simulink model "SLIPquadtrot"  (R2016a)
settings: Solver=ode45  StartTime=0.0  StopTime=10  MaxStep=1e-3  RelTol=1e-4  AbsTol=1e-6
values from neighbouring files (symbols this model uses):
  g = 9.81    [SLIPquad_params - Copy.m]    (also in SLIPquad_params.m; SLIPquad_paramswalk.m; purecmaes.m; purecmaeswalk.m)
  J = 4.58    [SLIPquad_params - Copy.m]    (also in SLIPquad_params.m; SLIPquad_paramswalk.m; purecmaes.m; purecmaeswalk.m)
  L = 0.5    [SLIPquad_params - Copy.m]    (also in SLIPquad_params.m; SLIPquad_paramswalk.m; purecmaes.m; purecmaeswalk.m)
  l0 = 1    [SLIPquad_params - Copy.m]    (also in SLIPquad_params.m; SLIPquad_paramswalk.m; purecmaes.m; purecmaeswalk.m)
  m = 80    [SLIPquad_params - Copy.m]    (also in SLIPquad_params.m; SLIPquad_paramswalk.m; purecmaes.m; purecmaeswalk.m)
  x0 = 0    [SLIPquad_params - Copy.m]    (also in SLIPquad_params.m; SLIPquad_paramswalk.m; purecmaes.m; purecmaeswalk.m)
  xrb0 = -l0*cos(a0br) + L*cos(t0)    [SLIPquad_params - Copy.m]    (also in SLIPquad_params.m)
  xrf0 = -l0*cos(a0fr) - L*cos(t0)    [SLIPquad_params - Copy.m]    (also in SLIPquad_params.m)
  y0 = 0.9730    (= 0.973)    [SLIPquad_params - Copy.m]    (also in SLIPquad_params.m = 0.9571; SLIPquad_paramswalk.m = x(6); purecmaes.m = 1; purecmaeswalk.m = x(6))
  yrb0 = l0*sin(a0br) + L*sin(t0)    [SLIPquad_params - Copy.m]    (also in SLIPquad_params.m)
  yrf0 = l0*sin(a0fr) - L*sin(t0)    [SLIPquad_params - Copy.m]    (also in SLIPquad_params.m)
libraries: simulink_extras x4, dspswit3 x1
settings Model: Creator=hgeyer  LastModifiedBy=Joe
settings DataIOCC: SaveFormat=Array  SignalLoggingSaveFormat=ModelDataLogs
settings OptimizationCC: ExpressionDepthLimit=2147483647
settings DebuggingCC: UnderspecifiedInitializationDetection=Classic  MergeDetectMultiDrivingBlocksExec=none  SolverPrmCheckMsg=warning  FcnCallInpInsideContextMsg=EnableAllAsWarning  AllowSymbolicDim=off  StateNameClashWarn=warning
settings HardwareCC: ProdBitPerPointer=32  ProdLargestAtomicFloat=None  ProdIntDivRoundTo=Undefined  ProdEndianess=Unspecified  ProdWordSize=32  ProdHWDeviceType=32-bit Generic
settings ModelReferenceCC: PropagateSignalLabelsOutOfModel=off
settings ConfigComp: CovModelRefEnable=Off

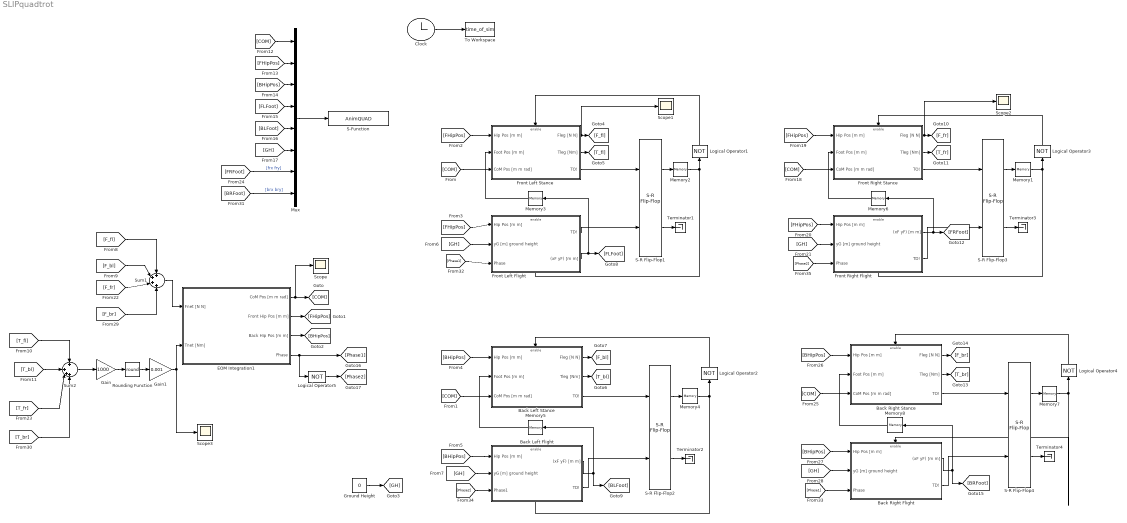
== system SLIPquadtrot ==
  Back Left Flight : Subsystem
  Back Left Stance : Subsystem
  Back Right Flight : Subsystem
  Back Right Stance : Subsystem
  Clock : Clock
      settings: Decimation=100
  EOM Integration1 : Subsystem
  Front Left Flight : Subsystem
  Front Left Stance : Subsystem
  Front Right Flight : Subsystem
  Front Right Stance : Subsystem
  Gain : Gain  Gain=1000
  Gain1 : Gain  Gain=0.001
  Ground Height : Constant  Value=0
  Logical Operator{1..5} (5 alike) : Logic  Operator=NOT  AllPortsSameDT=off  OutDataTypeStr=boolean
  Memory{1..2,4,7} (4 alike) : Memory  X0=1
  Memory3 : Memory  X0=[(x0 - xrf0) (y0 - yrf0) ]
  Memory5 : Memory  X0=[(x0 - xrb0) (y0 - yrb0)]
  Memory6 : Memory  X0=[(x0 - xrf0) (y0 - yrf0) ]
  Memory8 : Memory  X0=[(x0 - xrb0) (y0 - yrb0)]
  Mux : Mux  Inputs=8
  Rounding Function : Rounding  Operator=round
  S-Function : S-Function  FunctionName=AnimQUAD  Parameters=0.005  SFunctionDeploymentMode=off  EnableBusSupport=off
  S-R Flip-Flop{1..4} (4 alike) : simulink_extras/Flip Flops/S-R Flip-Flop  initial_condition=1
  Scope{,1..3} (4 alike) : Scope
  Sum1 : Sum  Inputs=++++
  Sum2 : Sum  Inputs=+|+++
  Terminator{1..4} (4 alike) : Terminator
  To Workspace : ToWorkspace  VariableName=time_of_sim  SampleTime=-1
      settings: MaxDataPoints=1
  wires:
  Front Left Stance/3(TO!) -> S-R Flip-Flop1/1
  S-R Flip-Flop1/1 -> Memory2/1
  Front Left Flight/1(TD!) -> S-R Flip-Flop1/2
  Memory2/1 -> Front Left Flight/Enable, Logical Operator1/1
  Logical Operator1/1 -> Front Left Stance/Enable
  S-R Flip-Flop1/2 -> Terminator1/1
  Front Left Flight/2((xF yF) [m m]) -> [FLFoot], Memory3/1
  Memory3/1 -> Front Left Stance/2(Foot Pos [m m])
  Back Left Stance/3(TO!) -> S-R Flip-Flop2/1
  S-R Flip-Flop2/1 -> Memory4/1
  Back Left Flight/2(TD!) -> S-R Flip-Flop2/2
  Memory4/1 -> Back Left Flight/Enable, Logical Operator2/1
  Logical Operator2/1 -> Back Left Stance/Enable
  S-R Flip-Flop2/2 -> Terminator2/1
  [GH] -> Back Left Flight/2(yG [m] ground height)
  Back Left Flight/1((xF yF) [m m]) -> [BLFoot], Memory5/1
  Memory5/1 -> Back Left Stance/2(Foot Pos [m m])
  Ground Height/1 -> [GH]
  [GH] -> Front Left Flight/2(yG [m] ground height)
  Front Left Stance/1(Fleg [N N]) -> Scope1/1, [F_fl]
  Front Left Stance/2(Tleg [Nm]) -> [T_fl]
  Back Left Stance/1(Fleg [N N]) -> [F_bl]
  Back Left Stance/2(Tleg [Nm]) -> [T_bl]
  [F_fl] -> Sum1/1
  [F_bl] -> Sum1/2
  [T_fl] -> Sum2/1
  [T_bl] -> Sum2/2
  Sum1/1 -> EOM Integration1/1(Fnet [N N])
  EOM Integration1/1(CoM Pos [m m rad]) -> Scope/1, [COM]
  EOM Integration1/2(Front Hip Pos [m m]) -> [FHipPos]
  EOM Integration1/3(Back Hip Pos [m m]) -> [BHipPos]
  [FHipPos] -> Front Left Stance/1(Hip Pos [m m])
  [FHipPos] -> Front Left Flight/1(Hip Pos [m m])
  [BHipPos] -> Back Left Stance/1(Hip Pos [m m])
  [BHipPos] -> Back Left Flight/1(Hip Pos [m m])
  [COM] -> Front Left Stance/3(CoM Pos [m m rad])
  [COM] -> Back Left Stance/3(CoM Pos [m m rad])
  Sum2/1 -> Gain/1
  Gain1/1 -> Scope3/1, EOM Integration1/2(Tnet [Nm])
  Gain/1 -> Rounding Function/1
  Rounding Function/1 -> Gain1/1
  Mux/1 -> S-Function/1
  [COM] -> Mux/1
  [FHipPos] -> Mux/2
  [BHipPos] -> Mux/3
  [FLFoot] -> Mux/4
  [BLFoot] -> Mux/5
  [GH] -> Mux/6
  [FRFoot] -> Mux/7  "[frx fry]"
  [BRFoot] -> Mux/8  "[brx bry]"
  Front Right Stance/3(TO!) -> S-R Flip-Flop3/1
  S-R Flip-Flop3/1 -> Memory1/1
  Front Right Flight/2(TD!) -> S-R Flip-Flop3/2
  Memory1/1 -> Front Right Flight/Enable, Logical Operator3/1
  Logical Operator3/1 -> Front Right Stance/Enable
  S-R Flip-Flop3/2 -> Terminator3/1
  Front Right Flight/1((xF yF) [m m]) -> Memory6/1, [FRFoot]
  Memory6/1 -> Front Right Stance/2(Foot Pos [m m])
  [GH] -> Front Right Flight/2(yG [m] ground height)
  Front Right Stance/1(Fleg [N N]) -> Scope2/1, [F_fr]
  Front Right Stance/2(Tleg [Nm]) -> [T_fr]
  [FHipPos] -> Front Right Stance/1(Hip Pos [m m])
  [FHipPos] -> Front Right Flight/1(Hip Pos [m m])
  [COM] -> Front Right Stance/3(CoM Pos [m m rad])
  [F_fr] -> Sum1/3
  [T_fr] -> Sum2/3
  Back Right Stance/3(TO!) -> S-R Flip-Flop4/1
  S-R Flip-Flop4/1 -> Memory7/1
  Back Right Flight/2(TD!) -> S-R Flip-Flop4/2
  Memory7/1 -> Back Right Flight/Enable, Logical Operator4/1
  Logical Operator4/1 -> Back Right Stance/Enable
  S-R Flip-Flop4/2 -> Terminator4/1
  [GH] -> Back Right Flight/2(yG [m] ground height)
  Back Right Flight/1((xF yF) [m m]) -> [BRFoot], Memory8/1
  Memory8/1 -> Back Right Stance/2(Foot Pos [m m])
  Back Right Stance/1(Fleg [N N]) -> [F_br]
  Back Right Stance/2(Tleg [Nm]) -> [T_br]
  [BHipPos] -> Back Right Stance/1(Hip Pos [m m])
  [BHipPos] -> Back Right Flight/1(Hip Pos [m m])
  [COM] -> Back Right Stance/3(CoM Pos [m m rad])
  [F_br] -> Sum1/4
  [T_br] -> Sum2/4
  Clock/1 -> To Workspace/1
  EOM Integration1/4(Phase) -> Logical Operator5/1, [Phase1]
  Logical Operator5/1 -> [Phase2]
  [Phase1] -> Front Left Flight/3(Phase)
  [Phase1] -> Back Right Flight/3(Phase)
  [Phase2] -> Back Left Flight/3(Phase1)
  [Phase2] -> Front Right Flight/3(Phase)

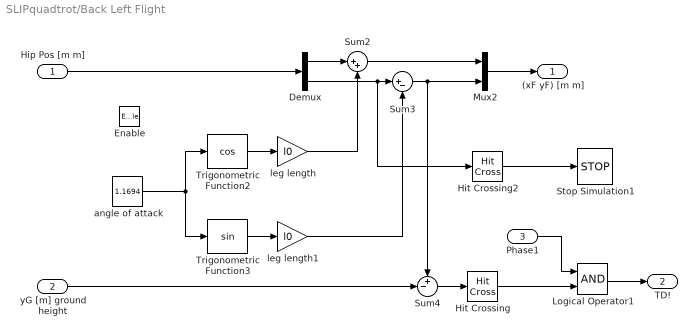
== system SLIPquadtrot/Back Left Flight ==
  Hip Pos [m m] : Inport
  yG [m] ground height : Inport  Port=2
  Phase1 : Inport  Port=3
  Enable : EnablePort  StatesWhenEnabling=reset
  Demux : Demux  Outputs=2
  Hit Crossing : HitCross  HitCrossingDirection=falling
  Hit Crossing2 : HitCross  HitCrossingOffset=-1  HitCrossingDirection=falling
  Logical Operator1 : Logic  AllPortsSameDT=off  OutDataTypeStr=boolean
  Mux2 : Mux  Inputs=2
  Stop Simulation1 : Stop
  Sum2 : Sum  Inputs=|++
  Sum3 : Sum  Inputs=|+-
  Sum4 : Sum  Inputs=+-|
  Trigonometric Function2 : Trigonometry  Operator=cos
  Trigonometric Function3 : Trigonometry
  angle of attack : Constant  Value=1.1694
  leg length : Gain  Gain=l0
  leg length1 : Gain  Gain=l0
  (xF yF) [m m] : Outport  InitialOutput=[0 0]
      settings: AttributesFormatString=%<OutputWhenDisabled>
  TD! : Outport  Port=2  OutputWhenDisabled=reset  InitialOutput=0
      settings: AttributesFormatString=%<OutputWhenDisabled>
  wires:
  Demux/2 -> Hit Crossing2/1, Sum3/1
  Demux/1 -> Sum2/1
  angle of attack/1 -> Trigonometric Function3/1, Trigonometric Function2/1
  Trigonometric Function2/1 -> leg length/1
  Trigonometric Function3/1 -> leg length1/1
  Hip Pos [m m]/1 -> Demux/1
  leg length/1 -> Sum2/2
  leg length1/1 -> Sum3/2
  Sum3/1 -> Mux2/2, Sum4/1
  Sum2/1 -> Mux2/1
  Mux2/1 -> (xF yF) [m m]/1
  yG [m] ground height/1 -> Sum4/2
  Sum4/1 -> Hit Crossing/1
  Hit Crossing2/1 -> Stop Simulation1/1
  Hit Crossing/1 -> Logical Operator1/2
  Phase1/1 -> Logical Operator1/1
  Logical Operator1/1 -> TD!/1

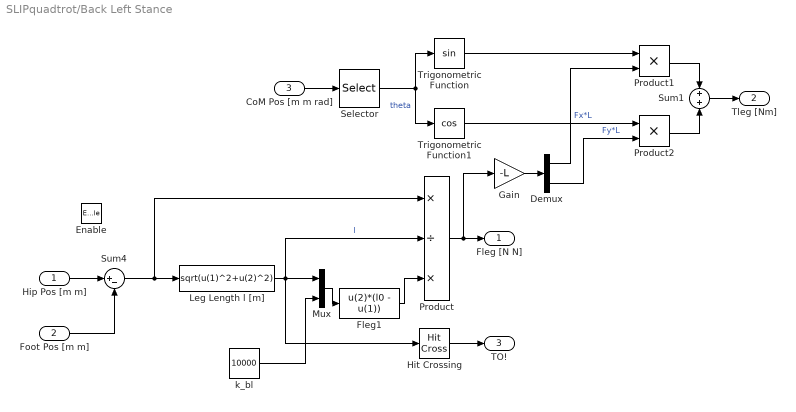
== system SLIPquadtrot/Back Left Stance ==
  Hip Pos [m m] : Inport
  Foot Pos [m m] : Inport  Port=2
  CoM Pos [m m rad] : Inport  Port=3
  Enable : EnablePort  StatesWhenEnabling=reset
  Demux : Demux  Outputs=2
  Fleg1 : Fcn  Expr=u(2)*(l0 - u(1))
  Gain : Gain  Gain=-L
  Hit Crossing : HitCross  HitCrossingOffset=l0  HitCrossingDirection=rising
  Leg Length l [m] : Fcn  Expr=sqrt(u(1)^2+u(2)^2)
  Mux : Mux  Inputs=2
  Product : Product  Inputs=*/*
  Product1 : Product
  Product2 : Product
  Selector : Selector  InputPortWidth=3  IndexOptions=Index vector (dialog)  Indices=[3]  OutputSizes=1
  Sum1 : Sum  Inputs=+|+
  Sum4 : Sum  Inputs=|+-
  Trigonometric Function : Trigonometry
  Trigonometric Function1 : Trigonometry  Operator=cos
  k_bl : Constant  Value=10000
  Fleg [N N] : Outport  OutputWhenDisabled=reset  InitialOutput=[0 0]
      settings: AttributesFormatString=%<OutputWhenDisabled>
  Tleg [Nm] : Outport  Port=2  OutputWhenDisabled=reset  InitialOutput=[0]
      settings: AttributesFormatString=%<OutputWhenDisabled>
  TO! : Outport  Port=3  OutputWhenDisabled=reset  InitialOutput=[0]
      settings: AttributesFormatString=%<OutputWhenDisabled>
  wires:
  Sum1/1 -> Tleg [Nm]/1
  Product1/1 -> Sum1/1
  Product2/1 -> Sum1/2
  Gain/1 -> Demux/1
  Demux/2 -> Product2/2  "Fy*L"
  Demux/1 -> Product1/2  "Fx*L"
  Trigonometric Function/1 -> Product1/1
  Trigonometric Function1/1 -> Product2/1
  Selector/1 -> Trigonometric Function/1, Trigonometric Function1/1  "theta"
  CoM Pos [m m rad]/1 -> Selector/1
  Foot Pos [m m]/1 -> Sum4/2
  Hip Pos [m m]/1 -> Sum4/1
  Hit Crossing/1 -> TO!/1
  Product/1 -> Fleg [N N]/1, Gain/1
  Fleg1/1 -> Product/3
  Leg Length l [m]/1 -> Hit Crossing/1, Mux/1, Product/2  "l"
  Sum4/1 -> Leg Length l [m]/1, Product/1
  Mux/1 -> Fleg1/1
  k_bl/1 -> Mux/2

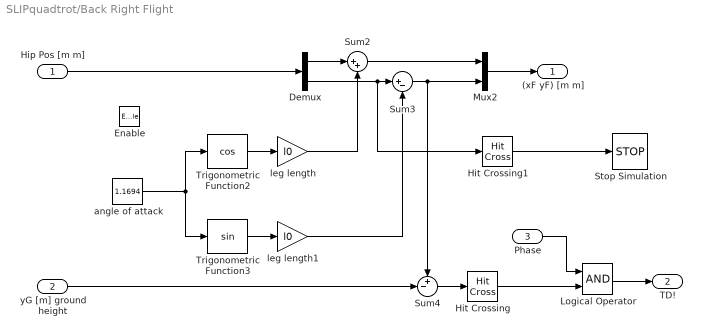
== system SLIPquadtrot/Back Right Flight ==
  Hip Pos [m m] : Inport
  yG [m] ground height : Inport  Port=2
  Phase : Inport  Port=3
  Enable : EnablePort  StatesWhenEnabling=reset
  Demux : Demux  Outputs=2
  Hit Crossing : HitCross  HitCrossingDirection=falling
  Hit Crossing1 : HitCross  HitCrossingOffset=-1  HitCrossingDirection=falling
  Logical Operator : Logic  AllPortsSameDT=off  OutDataTypeStr=boolean
  Mux2 : Mux  Inputs=2
  Stop Simulation : Stop
  Sum2 : Sum  Inputs=|++
  Sum3 : Sum  Inputs=|+-
  Sum4 : Sum  Inputs=+-|
  Trigonometric Function2 : Trigonometry  Operator=cos
  Trigonometric Function3 : Trigonometry
  angle of attack : Constant  Value=1.1694
  leg length : Gain  Gain=l0
  leg length1 : Gain  Gain=l0
  (xF yF) [m m] : Outport  InitialOutput=[0 0]
      settings: AttributesFormatString=%<OutputWhenDisabled>
  TD! : Outport  Port=2  OutputWhenDisabled=reset  InitialOutput=0
      settings: AttributesFormatString=%<OutputWhenDisabled>
  wires:
  Demux/2 -> Hit Crossing1/1, Sum3/1
  Demux/1 -> Sum2/1
  angle of attack/1 -> Trigonometric Function3/1, Trigonometric Function2/1
  Trigonometric Function2/1 -> leg length/1
  Trigonometric Function3/1 -> leg length1/1
  Hip Pos [m m]/1 -> Demux/1
  leg length/1 -> Sum2/2
  leg length1/1 -> Sum3/2
  Sum3/1 -> Mux2/2, Sum4/1
  Sum2/1 -> Mux2/1
  Mux2/1 -> (xF yF) [m m]/1
  yG [m] ground height/1 -> Sum4/2
  Sum4/1 -> Hit Crossing/1
  Hit Crossing1/1 -> Stop Simulation/1
  Hit Crossing/1 -> Logical Operator/2
  Phase/1 -> Logical Operator/1
  Logical Operator/1 -> TD!/1

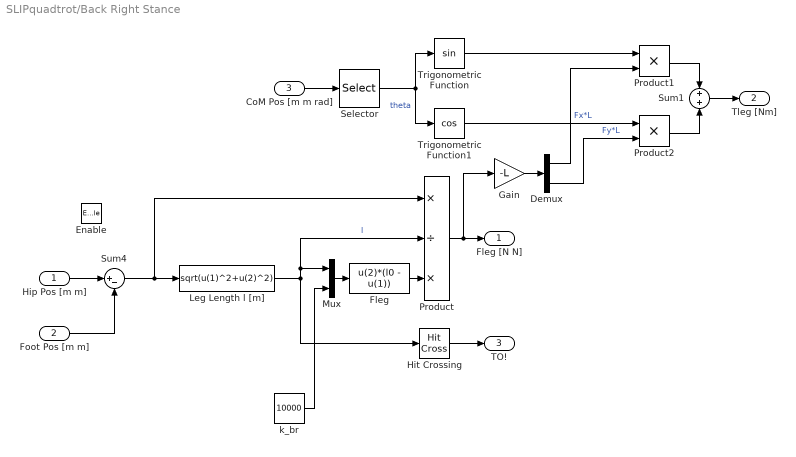
== system SLIPquadtrot/Back Right Stance ==
  Hip Pos [m m] : Inport
  Foot Pos [m m] : Inport  Port=2
  CoM Pos [m m rad] : Inport  Port=3
  Enable : EnablePort  StatesWhenEnabling=reset
  Demux : Demux  Outputs=2
  Fleg : Fcn  Expr=u(2)*(l0 - u(1))
  Gain : Gain  Gain=-L
  Hit Crossing : HitCross  HitCrossingOffset=l0  HitCrossingDirection=rising
  Leg Length l [m] : Fcn  Expr=sqrt(u(1)^2+u(2)^2)
  Mux : Mux  Inputs=2
  Product : Product  Inputs=*/*
  Product1 : Product
  Product2 : Product
  Selector : Selector  InputPortWidth=3  IndexOptions=Index vector (dialog)  Indices=[3]  OutputSizes=1
  Sum1 : Sum  Inputs=+|+
  Sum4 : Sum  Inputs=|+-
  Trigonometric Function : Trigonometry
  Trigonometric Function1 : Trigonometry  Operator=cos
  k_br : Constant  Value=10000
  Fleg [N N] : Outport  OutputWhenDisabled=reset  InitialOutput=[0 0]
      settings: AttributesFormatString=%<OutputWhenDisabled>
  Tleg [Nm] : Outport  Port=2  OutputWhenDisabled=reset  InitialOutput=[0]
      settings: AttributesFormatString=%<OutputWhenDisabled>
  TO! : Outport  Port=3  OutputWhenDisabled=reset  InitialOutput=[0]
      settings: AttributesFormatString=%<OutputWhenDisabled>
  wires:
  Sum1/1 -> Tleg [Nm]/1
  Product1/1 -> Sum1/1
  Product2/1 -> Sum1/2
  Gain/1 -> Demux/1
  Demux/2 -> Product2/2  "Fy*L"
  Demux/1 -> Product1/2  "Fx*L"
  Trigonometric Function/1 -> Product1/1
  Trigonometric Function1/1 -> Product2/1
  Selector/1 -> Trigonometric Function/1, Trigonometric Function1/1  "theta"
  CoM Pos [m m rad]/1 -> Selector/1
  Foot Pos [m m]/1 -> Sum4/2
  Hip Pos [m m]/1 -> Sum4/1
  Hit Crossing/1 -> TO!/1
  Product/1 -> Fleg [N N]/1, Gain/1
  Fleg/1 -> Product/3
  Leg Length l [m]/1 -> Mux/1, Product/2, Hit Crossing/1  "l"
  Sum4/1 -> Leg Length l [m]/1, Product/1
  Mux/1 -> Fleg/1
  k_br/1 -> Mux/2

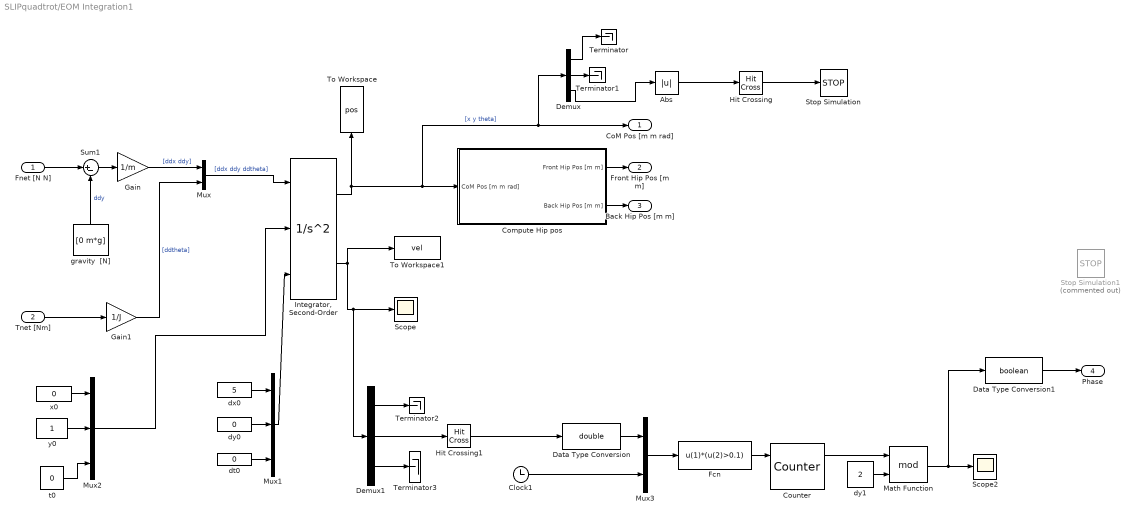
== system SLIPquadtrot/EOM Integration1 ==
  Fnet [N N] : Inport
  Tnet [Nm] : Inport  Port=2
  Abs : Abs
  Clock1 : Clock
  Compute Hip pos : Subsystem
  Counter : dspswit3/Counter  Direction=Up  CountEvent=Rising edge  CounterSize=User defined  MaxCount=255  InitialCount=0  Output=Count and Hit  HitValue=32  ResetInput=on  SamplesPerFrame=1  Ts=1  CntDtype=double  HitDtype=Logical
  Data Type Conversion : DataTypeConversion  OutDataTypeStr=double
  Data Type Conversion1 : DataTypeConversion  OutDataTypeStr=boolean
  Demux : Demux  Outputs=3
  Demux1 : Demux  Outputs=3
  Fcn : Fcn  Expr=u(1)*(u(2)>0.1)
  Gain : Gain  Gain=1/m
  Gain1 : Gain  Gain=1/J
  Hit Crossing : HitCross  HitCrossingOffset=1.57
  Hit Crossing1 : HitCross  HitCrossingOffset=0.0001  HitCrossingDirection=falling
  "Integrator, Second-Order" : SecondOrderIntegrator  ICSourceX=external  ICSourceDXDT=external
  Math Function : Math  Operator=mod  SaturateOnIntegerOverflow=on
  Mux : Mux  Inputs=2
  Mux1 : Mux  Inputs=3
  Mux2 : Mux  Inputs=3
  Mux3 : Mux  Inputs=2
  Scope : Scope
  Scope2 : Scope
  Stop Simulation : Stop
  Stop Simulation1 : Stop  Commented=on
  Sum1 : Sum  Inputs=|+-
  Terminator{,1..3} (4 alike) : Terminator
  To Workspace : ToWorkspace  VariableName=pos  SampleTime=-1
  To Workspace1 : ToWorkspace  VariableName=vel  SampleTime=-1
  dt0 : Constant  Value=0
  dx0 : Constant  Value=5
  dy0 : Constant  Value=0
  dy1 : Constant  Value=2
  gravity  [N] : Constant  Value=[0 m*g]
  t0 : Constant  Value=0
  x0 : Constant  Value=0
  y0 : Constant
  CoM Pos [m m rad] : Outport
  Front Hip Pos [m m] : Outport  Port=2
  Back Hip Pos [m m] : Outport  Port=3
  Phase : Outport  Port=4
  wires:
  Compute Hip pos/1(Front Hip Pos [m m]) -> Front Hip Pos [m m]/1
  "Integrator, Second-Order"/1 -> To Workspace/1, Demux/1, CoM Pos [m m rad]/1, Compute Hip pos/1(CoM Pos [m m rad])  "[x y theta]"
  Tnet [Nm]/1 -> Gain1/1
  Gain1/1 -> Mux/2  "[ddtheta]"
  Mux/1 -> "Integrator, Second-Order"/1  "[ddx ddy ddtheta]"
  Fnet [N N]/1 -> Sum1/1
  Gain/1 -> Mux/1  "[ddx ddy]"
  Mux2/1 -> "Integrator, Second-Order"/2
  gravity  [N]/1 -> Sum1/2  "ddy"
  Sum1/1 -> Gain/1
  Compute Hip pos/2(Back Hip Pos [m m]) -> Back Hip Pos [m m]/1
  Mux1/1 -> "Integrator, Second-Order"/3
  dx0/1 -> Mux1/1
  dy0/1 -> Mux1/2
  dt0/1 -> Mux1/3
  Demux/3 -> Abs/1
  Demux/1 -> Terminator/1
  Demux/2 -> Terminator1/1
  Hit Crossing/1 -> Stop Simulation/1
  Abs/1 -> Hit Crossing/1
  Hit Crossing1/1 -> Data Type Conversion/1
  "Integrator, Second-Order"/2 -> To Workspace1/1, Demux1/1, Scope/1
  Demux1/3 -> Terminator3/1
  x0/1 -> Mux2/1
  y0/1 -> Mux2/2
  t0/1 -> Mux2/3
  Demux1/2 -> Hit Crossing1/1
  Demux1/1 -> Terminator2/1
  Clock1/1 -> Mux3/2
  Mux3/1 -> Fcn/1
  Data Type Conversion/1 -> Mux3/1
  Fcn/1 -> Counter/1
  Counter/1 -> Math Function/1
  dy1/1 -> Math Function/2
  Math Function/1 -> Data Type Conversion1/1, Scope2/1
  Data Type Conversion1/1 -> Phase/1

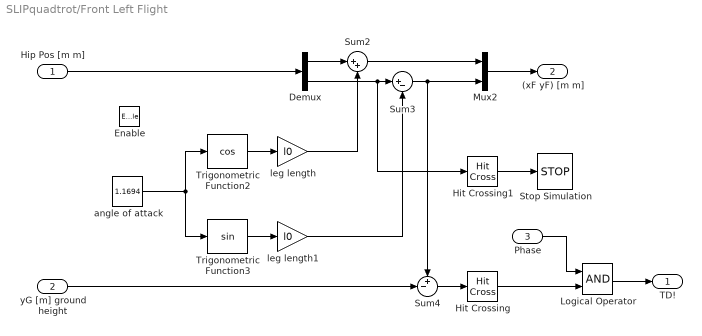
== system SLIPquadtrot/Front Left Flight ==
  Hip Pos [m m] : Inport
  yG [m] ground height : Inport  Port=2
  Phase : Inport  Port=3
  Enable : EnablePort  StatesWhenEnabling=reset
  Demux : Demux  Outputs=2
  Hit Crossing : HitCross  HitCrossingDirection=falling
  Hit Crossing1 : HitCross  HitCrossingOffset=-1  HitCrossingDirection=falling
  Logical Operator : Logic  AllPortsSameDT=off  OutDataTypeStr=boolean
  Mux2 : Mux  Inputs=2
  Stop Simulation : Stop
  Sum2 : Sum  Inputs=|++
  Sum3 : Sum  Inputs=|+-
  Sum4 : Sum  Inputs=+-|
  Trigonometric Function2 : Trigonometry  Operator=cos
  Trigonometric Function3 : Trigonometry
  angle of attack : Constant  Value=1.1694
  leg length : Gain  Gain=l0
  leg length1 : Gain  Gain=l0
  TD! : Outport  OutputWhenDisabled=reset  InitialOutput=0
      settings: AttributesFormatString=%<OutputWhenDisabled>
  (xF yF) [m m] : Outport  Port=2  InitialOutput=[0 0]
      settings: AttributesFormatString=%<OutputWhenDisabled>
  wires:
  Hit Crossing1/1 -> Stop Simulation/1
  Sum4/1 -> Hit Crossing/1
  yG [m] ground height/1 -> Sum4/2
  Mux2/1 -> (xF yF) [m m]/1
  Sum2/1 -> Mux2/1
  Sum3/1 -> Sum4/1, Mux2/2
  leg length1/1 -> Sum3/2
  leg length/1 -> Sum2/2
  Hip Pos [m m]/1 -> Demux/1
  Trigonometric Function3/1 -> leg length1/1
  Trigonometric Function2/1 -> leg length/1
  angle of attack/1 -> Trigonometric Function2/1, Trigonometric Function3/1
  Demux/1 -> Sum2/1
  Demux/2 -> Sum3/1, Hit Crossing1/1
  Hit Crossing/1 -> Logical Operator/2
  Phase/1 -> Logical Operator/1
  Logical Operator/1 -> TD!/1

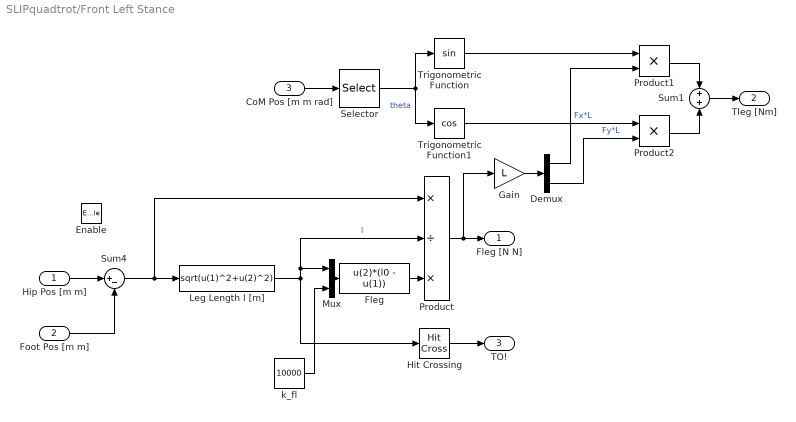
== system SLIPquadtrot/Front Left Stance ==
  Hip Pos [m m] : Inport
  Foot Pos [m m] : Inport  Port=2
  CoM Pos [m m rad] : Inport  Port=3
  Enable : EnablePort  StatesWhenEnabling=reset
  Demux : Demux  Outputs=2
  Fleg : Fcn  Expr=u(2)*(l0 - u(1))
  Gain : Gain  Gain=L
  Hit Crossing : HitCross  HitCrossingOffset=l0  HitCrossingDirection=rising
  Leg Length l [m] : Fcn  Expr=sqrt(u(1)^2+u(2)^2)
  Mux : Mux  Inputs=2
  Product : Product  Inputs=*/*
  Product1 : Product
  Product2 : Product
  Selector : Selector  InputPortWidth=3  IndexOptions=Index vector (dialog)  Indices=[3]  OutputSizes=1
  Sum1 : Sum  Inputs=+|+
  Sum4 : Sum  Inputs=|+-
  Trigonometric Function : Trigonometry
  Trigonometric Function1 : Trigonometry  Operator=cos
  k_fl : Constant  Value=10000
  Fleg [N N] : Outport  OutputWhenDisabled=reset  InitialOutput=[0 0]
      settings: AttributesFormatString=%<OutputWhenDisabled>
  Tleg [Nm] : Outport  Port=2  OutputWhenDisabled=reset  InitialOutput=[0]
      settings: AttributesFormatString=%<OutputWhenDisabled>
  TO! : Outport  Port=3  OutputWhenDisabled=reset  InitialOutput=[0]
      settings: AttributesFormatString=%<OutputWhenDisabled>
  wires:
  Sum4/1 -> Product/1, Leg Length l [m]/1
  Leg Length l [m]/1 -> Mux/1, Product/2, Hit Crossing/1  "l"
  Fleg/1 -> Product/3
  Product/1 -> Gain/1, Fleg [N N]/1
  Hit Crossing/1 -> TO!/1
  Hip Pos [m m]/1 -> Sum4/1
  Foot Pos [m m]/1 -> Sum4/2
  CoM Pos [m m rad]/1 -> Selector/1
  Selector/1 -> Trigonometric Function1/1, Trigonometric Function/1  "theta"
  Trigonometric Function1/1 -> Product2/1
  Trigonometric Function/1 -> Product1/1
  Demux/1 -> Product1/2  "Fx*L"
  Demux/2 -> Product2/2  "Fy*L"
  Gain/1 -> Demux/1
  Product2/1 -> Sum1/2
  Product1/1 -> Sum1/1
  Sum1/1 -> Tleg [Nm]/1
  Mux/1 -> Fleg/1
  k_fl/1 -> Mux/2

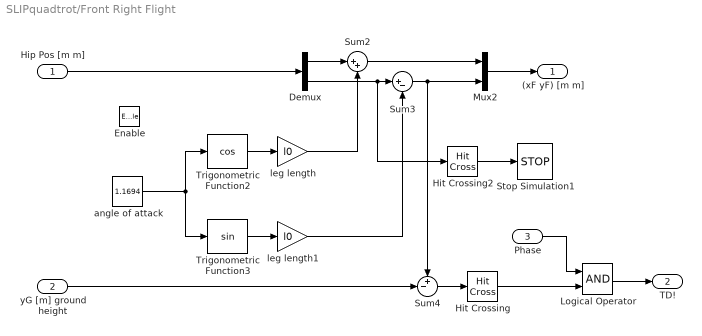
== system SLIPquadtrot/Front Right Flight ==
  Hip Pos [m m] : Inport
  yG [m] ground height : Inport  Port=2
  Phase : Inport  Port=3
  Enable : EnablePort  StatesWhenEnabling=reset
  Demux : Demux  Outputs=2
  Hit Crossing : HitCross  HitCrossingDirection=falling
  Hit Crossing2 : HitCross  HitCrossingOffset=-1  HitCrossingDirection=falling
  Logical Operator : Logic  AllPortsSameDT=off  OutDataTypeStr=boolean
  Mux2 : Mux  Inputs=2
  Stop Simulation1 : Stop
  Sum2 : Sum  Inputs=|++
  Sum3 : Sum  Inputs=|+-
  Sum4 : Sum  Inputs=+-|
  Trigonometric Function2 : Trigonometry  Operator=cos
  Trigonometric Function3 : Trigonometry
  angle of attack : Constant  Value=1.1694
  leg length : Gain  Gain=l0
  leg length1 : Gain  Gain=l0
  (xF yF) [m m] : Outport  InitialOutput=[0 0]
      settings: AttributesFormatString=%<OutputWhenDisabled>
  TD! : Outport  Port=2  OutputWhenDisabled=reset  InitialOutput=0
      settings: AttributesFormatString=%<OutputWhenDisabled>
  wires:
  Sum4/1 -> Hit Crossing/1
  yG [m] ground height/1 -> Sum4/2
  Mux2/1 -> (xF yF) [m m]/1
  Sum2/1 -> Mux2/1
  Sum3/1 -> Sum4/1, Mux2/2
  leg length1/1 -> Sum3/2
  leg length/1 -> Sum2/2
  Hip Pos [m m]/1 -> Demux/1
  Trigonometric Function3/1 -> leg length1/1
  Trigonometric Function2/1 -> leg length/1
  angle of attack/1 -> Trigonometric Function2/1, Trigonometric Function3/1
  Demux/1 -> Sum2/1
  Demux/2 -> Hit Crossing2/1, Sum3/1
  Hit Crossing2/1 -> Stop Simulation1/1
  Hit Crossing/1 -> Logical Operator/2
  Phase/1 -> Logical Operator/1
  Logical Operator/1 -> TD!/1

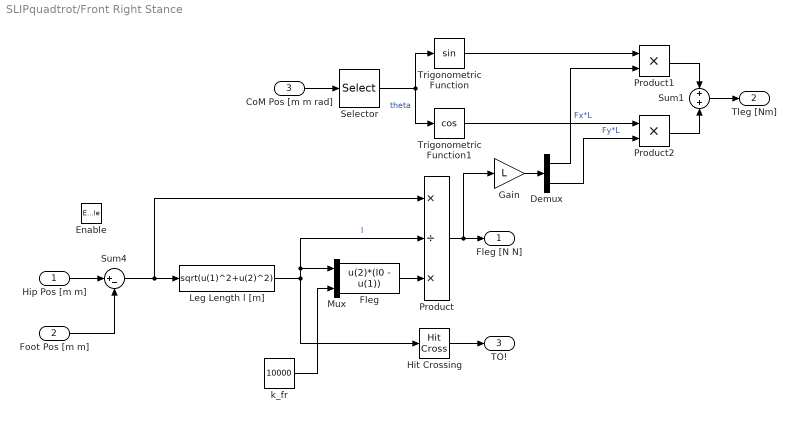
== system SLIPquadtrot/Front Right Stance ==
  Hip Pos [m m] : Inport
  Foot Pos [m m] : Inport  Port=2
  CoM Pos [m m rad] : Inport  Port=3
  Enable : EnablePort  StatesWhenEnabling=reset
  Demux : Demux  Outputs=2
  Fleg : Fcn  Expr=u(2)*(l0 - u(1))
  Gain : Gain  Gain=L
  Hit Crossing : HitCross  HitCrossingOffset=l0  HitCrossingDirection=rising
  Leg Length l [m] : Fcn  Expr=sqrt(u(1)^2+u(2)^2)
  Mux : Mux  Inputs=2
  Product : Product  Inputs=*/*
  Product1 : Product
  Product2 : Product
  Selector : Selector  InputPortWidth=3  IndexOptions=Index vector (dialog)  Indices=[3]  OutputSizes=1
  Sum1 : Sum  Inputs=+|+
  Sum4 : Sum  Inputs=|+-
  Trigonometric Function : Trigonometry
  Trigonometric Function1 : Trigonometry  Operator=cos
  k_fr : Constant  Value=10000
  Fleg [N N] : Outport  OutputWhenDisabled=reset  InitialOutput=[0 0]
      settings: AttributesFormatString=%<OutputWhenDisabled>
  Tleg [Nm] : Outport  Port=2  OutputWhenDisabled=reset  InitialOutput=[0]
      settings: AttributesFormatString=%<OutputWhenDisabled>
  TO! : Outport  Port=3  OutputWhenDisabled=reset  InitialOutput=[0]
      settings: AttributesFormatString=%<OutputWhenDisabled>
  wires:
  Sum4/1 -> Product/1, Leg Length l [m]/1
  Leg Length l [m]/1 -> Mux/1, Product/2, Hit Crossing/1  "l"
  Fleg/1 -> Product/3
  Product/1 -> Gain/1, Fleg [N N]/1
  Hit Crossing/1 -> TO!/1
  Hip Pos [m m]/1 -> Sum4/1
  Foot Pos [m m]/1 -> Sum4/2
  CoM Pos [m m rad]/1 -> Selector/1
  Selector/1 -> Trigonometric Function1/1, Trigonometric Function/1  "theta"
  Trigonometric Function1/1 -> Product2/1
  Trigonometric Function/1 -> Product1/1
  Demux/1 -> Product1/2  "Fx*L"
  Demux/2 -> Product2/2  "Fy*L"
  Gain/1 -> Demux/1
  Product2/1 -> Sum1/2
  Product1/1 -> Sum1/1
  Sum1/1 -> Tleg [Nm]/1
  Mux/1 -> Fleg/1
  k_fr/1 -> Mux/2

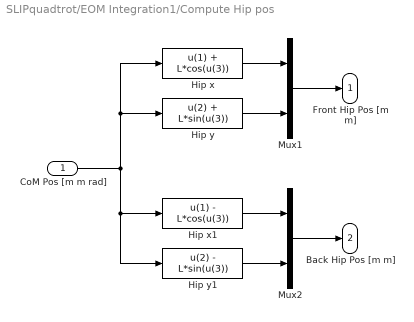
== system SLIPquadtrot/EOM Integration1/Compute Hip pos ==
  CoM Pos [m m rad] : Inport
  Hip x : Fcn  Expr=u(1) + L*cos(u(3))
  Hip x1 : Fcn  Expr=u(1) - L*cos(u(3))
  Hip y : Fcn  Expr=u(2) + L*sin(u(3))
  Hip y1 : Fcn  Expr=u(2) - L*sin(u(3))
  Mux1 : Mux  Inputs=2
  Mux2 : Mux  Inputs=2
  Front Hip Pos [m m] : Outport
  Back Hip Pos [m m] : Outport  Port=2
  wires:
  Hip y/1 -> Mux1/2
  Mux1/1 -> Front Hip Pos [m m]/1
  Hip x/1 -> Mux1/1
  Hip y1/1 -> Mux2/2
  Mux2/1 -> Back Hip Pos [m m]/1
  Hip x1/1 -> Mux2/1
  CoM Pos [m m rad]/1 -> Hip x/1, Hip y/1, Hip y1/1, Hip x1/1
